simulink model "EKF_SIL_02_newdelIpsOOSM"  (R2015a)
settings: Solver=ode45  StartTime=0.0  StopTime=50  RelTol=1e-3
model workspace: external: MATLAB File InitOOSM.m (data not in the file)
values from neighbouring files (symbols this model uses):
  Cov_nu = [0.005 0 0 0 ... (first row only)    [InitOOSM.m]    (also in InitSIL.m; Init_Model_02_Simulink.m; Init_Model_02_Simulink_SIL1.m)
  Cov_r = [0.003 0 0 ... (first row only)    [InitOOSM.m]    (also in InitSIL.m; Init_Model_02_Simulink.m; Init_Model_02_Simulink_SIL1.m)
  e_force_x = 0    [InitOOSM.m]    (also in InitSIL.m; Init_Model_02_Simulink.m; Init_Model_02_Simulink_SIL1.m)
  e_force_y = 0    [InitOOSM.m]    (also in InitSIL.m; Init_Model_02_Simulink.m; Init_Model_02_Simulink_SIL1.m)
  e_force_z = 0    [InitOOSM.m]    (also in InitSIL.m; Init_Model_02_Simulink.m; Init_Model_02_Simulink_SIL1.m)
  ieps = [-0.7071;0;0;0.7071]    [InitOOSM.m]    (also in InitSIL.m; Init_Model_02_Simulink.m = [-0.7071; 0; 0; 0.7071]; Init_Model_02_Simulink_SIL1.m)
  ita = [0.5;0.5;0.5;0.5]    [InitOOSM.m]    (also in InitSIL.m; Init_Model_02_Simulink.m = [0.5; 0.5; 0.5; 0.5]; Init_Model_02_Simulink_SIL1.m)
  n = 0.00    (= 0)    [InitOOSM.m]    (also in InitSIL.m; Init_Model_02_Simulink.m; Init_Model_02_Simulink_SIL1.m)
  P_0 = 0.5*eye(18,18)    [InitOOSM.m]    (also in InitSIL.m = 0.05*eye(12,12); Init_Model_02_Simulink.m = 0.005*eye(12,12); Init_Model_02_Simulink_SIL1.m = 0.005*eye(12,12))
  P_k = Simulink.Signal    [InitOOSM.m]    (also in InitSIL.m; Init_Model_02_Simulink.m; Init_Model_02_Simulink_SIL1.m)
  p_x = 0.75    [InitOOSM.m]    (also in InitSIL.m; Init_Model_02_Simulink.m; Init_Model_02_Simulink_SIL1.m)
  p_y = 0.125    [InitOOSM.m]    (also in InitSIL.m; Init_Model_02_Simulink.m; Init_Model_02_Simulink_SIL1.m)
  p_z = -0.8    [InitOOSM.m]    (also in InitSIL.m; Init_Model_02_Simulink.m; Init_Model_02_Simulink_SIL1.m)
  parameter_gravitation = 3.986005E+14    (= 398600500000000)    [InitOOSM.m]    (also in InitSIL.m; Init_Model_02_Simulink.m; Init_Model_02_Simulink_SIL1.m)
  rho = [0.04;0;0.3]    [InitOOSM.m]    (also in InitSIL.m; Init_Model_02_Simulink.m = [0.04; 0; 0.3]; Init_Model_02_Simulink_SIL1.m)
  rho_c = [-0.00017;   -0.9780;   -0.1854]    [InitOOSM.m]    (also in InitSIL.m = [0.00036;   -0.9865;   -0.1854]; Init_Model_02_Simulink.m = [0.00036; -0.9865; -0.1854]; Init_Model_02_Simulink_SIL1.m = [0.00036;   -0.9865;   -0.1854])
  sig_f = 2E-6    (= 2e-06)    [InitOOSM.m]    (also in InitSIL.m; Init_Model_02_Simulink.m; Init_Model_02_Simulink_SIL1.m)
  sig_tau = 2.5E-5    (= 2.5e-05)    [InitOOSM.m]    (also in InitSIL.m; Init_Model_02_Simulink.m; Init_Model_02_Simulink_SIL1.m)
  t_delta = 0.2    [InitOOSM.m]    (also in InitSIL.m; Init_Model_02_Simulink.m; Init_Model_02_Simulink_SIL1.m)
  t_Kalman = 0.01    [InitOOSM.m]    (also in InitSIL.m; Init_Model_02_Simulink.m; Init_Model_02_Simulink_SIL1.m)
  t_RobotSense = 0.05    [InitOOSM.m]    (also in InitSIL.m; Init_Model_02_Simulink.m; Init_Model_02_Simulink_SIL1.m)
  tau_1 = 0    [InitOOSM.m]    (also in InitSIL.m; Init_Model_02_Simulink.m; Init_Model_02_Simulink_SIL1.m)
  tau_2 = 0    [InitOOSM.m]    (also in InitSIL.m; Init_Model_02_Simulink.m; Init_Model_02_Simulink_SIL1.m)
  tau_3 = 0    [InitOOSM.m]    (also in InitSIL.m; Init_Model_02_Simulink.m; Init_Model_02_Simulink_SIL1.m)
  U_n_d = Simulink.Signal    [InitOOSM.m]    (also in InitSIL.m; Init_Model_02_Simulink.m; Init_Model_02_Simulink_SIL1.m)
  X_a_0 = [0; 0; 0; 1; 0; 0; 0; 0; 0; 0; 0; 0; 0;0;0;0;0;0;0;1]    [InitOOSM.m]    (also in InitSIL.m = [0; 0; 0; 1; 0; 0; 0; 0; 0; 0; 0; 0; 0]; Init_Model_02_Simulink.m = [0;0;0;0.707000000000000;0.707000000000000;0.200000000000000; Init_Model_02_Simulink_SIL1.m = [0;0;0.707;0.707;0.2;-0.02;0.0001;0.02;-1.80;0.50;-0.05;0.00)
  x_k = Simulink.Signal    [InitOOSM.m]    (also in InitSIL.m; Init_Model_02_Simulink.m; Init_Model_02_Simulink_SIL1.m)
libraries: simulink x9, dspmtrx3 x4, aerolibtransform2 x2, visionsinks x1
(part 2 of 6)

== system EKF_SIL_02_newdelIpsOOSM/EKF/OOSM_KF ==
  "trig_cap " : Inport
  P_pre : Inport  Port=2
  X_a_\(k) : Inport  Port=3
  V : Inport  Port=4
  trig_meas : Inport  Port=5
  ts_meas : Inport  Port=6
  " X_d1" : Inport  Port=7
  " X_d2" : Inport  Port=8
  " X_d3" : Inport  Port=9
  Constant : Constant  Value=0
  IC : InitialCondition  Value=0
  IC1 : InitialCondition  Value=0
  OOSM_KF : Subsystem
  OOSM_enable : Subsystem
  Scope : Scope
      settings: YMin=0  YMax=1  SaveName=ScopeData7
  Scope1 : Scope
      settings: YMin=0  YMax=1  SaveName=ScopeData34
  Selector : Selector  InputPortWidth=6  Indices=[4:6]
  Subsystem : Subsystem
  U_n_d : Outport
  x_d : Outport  Port=2
  P_d : Outport  Port=3
  UF : Outport  Port=4
  Phi : Outport  Port=5
  OOSM_trig : Outport  Port=6
  wires:
  "trig_cap "/1 -> OOSM_enable/1("trig_cap ")
  Constant/1 -> OOSM_KF/1(del_t)
  OOSM_enable/2(reset_trigger) -> IC1/1
  IC1/1 -> OOSM_KF/2(reset_trigger)
  OOSM_enable/3("q_nominal ") -> OOSM_KF/3(q_nominal)
  OOSM_KF/1(U_n_d) -> U_n_d/1
  OOSM_KF/2(x_d) -> x_d/1
  OOSM_KF/3(P_d) -> P_d/1
  P_pre/1 -> OOSM_KF/4(P_pre(k))
  Subsystem/1(X_a(k+1)) -> OOSM_KF/5("x(k) ")
  V/1 -> Selector/1, OOSM_KF/6(V), Subsystem/2(V)
  OOSM_enable/4(ieps_nominal_out) -> OOSM_KF/7(ieps_nominal)
  OOSM_KF/4(UF) -> UF/1
  OOSM_KF/5(Phi) -> Phi/1
  trig_meas/1 -> OOSM_enable/2(trig_meas)
  OOSM_enable/1(Trigger) -> IC/1
  Selector/1 -> OOSM_enable/3(omega_robot)
  OOSM_enable/5(OOSM_trig) -> Scope1/1, OOSM_trig/1
  ts_meas/1 -> OOSM_enable/4(ts_meas)
  X_a_\(k)/1 -> Subsystem/1(X_a)
  IC/1 -> OOSM_KF/Enable, Scope/1
  " X_d1"/1 -> OOSM_KF/8(" X_d1")
  " X_d2"/1 -> OOSM_KF/9(" X_d2")
  " X_d3"/1 -> OOSM_KF/10(" X_d3")

== system EKF_SIL_02_newdelIpsOOSM/EKF/Predictor ==
  X_a(K) : Inport
  P_previous(k) : Inport  Port=2
  trigger : Inport  Port=3
  V : Inport  Port=4
  Create Bus [State Vector,X_a] : Subsystem
  Create Bus [State Vector,X_a]1 : Subsystem
  Create State error covariance (P) : Subsystem
  Delay : Delay  DelayLength=1  InitialCondition=0
  Display : Display
  Integrator : Subsystem
  X_a(k+1) : Outport
  P_current(k+1) : Outport  Port=2
  wires:
  Create Bus [State Vector,X_a]1/1(X_bus) -> Create State error covariance (P)/1(X_a)
  Create State error covariance (P)/1(P_current) -> P_current(k+1)/1
  P_previous(k)/1 -> Create State error covariance (P)/2(P_previous)
  trigger/1 -> Delay/1
  V/1 -> Create State error covariance (P)/3(V), Integrator/2(V)
  X_a(K)/1 -> Create Bus [State Vector,X_a]1/1(X), Integrator/1(X_a)
  Create Bus [State Vector,X_a]/1(X_bus) -> Display/1, X_a(k+1)/1
  Integrator/1(X_a(k+1)) -> Create Bus [State Vector,X_a]/1(X)

== system EKF_SIL_02_newdelIpsOOSM/EKF/Trigger logic ==
  timestamp_target : Inport
  meas : Inport  Port=2
  timestamp_robot : Inport  Port=3
  Bus Selector : BusSelector  OutputSignals=r_c,Mu
  Bus Selector1 : BusSelector  OutputSignals=rho_c,ieps
  Compare To Zero1 : simulink/Logic and Bit Operations/Compare To Zero  relop=>  OutDataTypeStr=boolean
  Compare To Zero2 : simulink/Logic and Bit Operations/Compare To Zero  relop=>  OutDataTypeStr=boolean
  Detect Increase : simulink/Logic and Bit Operations/Detect Increase  vinit=0  InputProcessing=Inherited  OutDataTypeStr=boolean
  Detect Increase1 : simulink/Logic and Bit Operations/Detect Increase  vinit=0  InputProcessing=Inherited  OutDataTypeStr=boolean
  Dot Product1 : DotProduct  InputSameDT=on  OutDataTypeStr=Inherit: Inherit via internal rule
  Dot Product2 : DotProduct  InputSameDT=on  OutDataTypeStr=Inherit: Inherit via internal rule
  Logical Operator1 : Logic  AllPortsSameDT=off  OutDataTypeStr=boolean
  Logical Operator2 : Logic  Operator=OR  AllPortsSameDT=off  OutDataTypeStr=boolean
  Logical Operator3 : Logic  AllPortsSameDT=off  OutDataTypeStr=boolean
  Math Function1 : Math  Operator=transpose  SaturateOnIntegerOverflow=on
  Math Function2 : Math  Operator=transpose  SaturateOnIntegerOverflow=on
  Mux : Mux  Inputs=2
  Mux1 : Mux  Inputs=2
  Scope : Scope
      settings: YMin=0  YMax=1  SaveName=ScopeData32
  "Trigger " : Outport
  "Trigger_1 " : Outport  Port=2
  "Trigger_2 " : Outport  Port=3
  ts_meas : Outport  Port=4
  wires:
  meas/1 -> Bus Selector1/1, Bus Selector/1
  Bus Selector/1 -> Mux/1  "<r_c>"
  Bus Selector/2 -> Mux/2  "<Mu>"
  Bus Selector1/1 -> Mux1/1  "<rho_c>"
  Bus Selector1/2 -> Mux1/2  "<ieps>"
  Math Function1/1 -> Dot Product1/2
  Mux/1 -> Dot Product1/1, Math Function1/1
  Mux1/1 -> Dot Product2/1, Math Function2/1
  Math Function2/1 -> Dot Product2/2
  Dot Product1/1 -> Compare To Zero1/1
  Dot Product2/1 -> Compare To Zero2/1
  Compare To Zero1/1 -> Logical Operator1/1
  timestamp_robot/1 -> Detect Increase1/1
  Detect Increase/1 -> Logical Operator1/2
  Detect Increase1/1 -> Logical Operator3/2
  Compare To Zero2/1 -> Logical Operator3/1
  Logical Operator3/1 -> Logical Operator2/2, "Trigger_2 "/1
  timestamp_target/1 -> ts_meas/1, Detect Increase/1
  Logical Operator2/1 -> Scope/1, "Trigger "/1
  Logical Operator1/1 -> Logical Operator2/1, "Trigger_1 "/1

== system EKF_SIL_02_newdelIpsOOSM/Plant/Dynamic Model (Differential equations) ==
  X_a(t) : Inport
  Bus Creator : BusCreator
  Constant : Constant  Value=[0]
  Constant1 : Constant  Value=zeros(3,1)
  "Orbital Dynamics " : Subsystem
  Quaternion Kinematics : Subsystem
  Rotational Dynamics : Subsystem
  Vector Concatenate : Concatenate
  n : Constant  Value=n
  omega : Selector  NumberOfDimensions=2  InputPortWidth=3  IndexOptions=Index vector (dialog),Index vector (dialog)  Indices=[5 6 7],1  OutputSizes=1,1
  p : Constant  Value=[p_x;p_y;p_z]
  parameter_gravitation : Constant  Value=parameter_gravitation
  q : Selector  NumberOfDimensions=2  InputPortWidth=3  IndexOptions=Index vector (dialog),Index vector (dialog)  Indices=[1 2 3 4],1  OutputSizes=1,1
  r : Selector  NumberOfDimensions=2  InputPortWidth=3  IndexOptions=Index vector (dialog),Index vector (dialog)  Indices=[8 9 10],1  OutputSizes=1,1
  r_dot : Selector  NumberOfDimensions=2  InputPortWidth=3  IndexOptions=Index vector (dialog),Index vector (dialog)  Indices=[11 12 13],1  OutputSizes=1,1
  X_a(t+1) : Outport
  wires:
  Constant/1 -> Vector Concatenate/2
  p/1 -> Rotational Dynamics/2(p)
  Vector Concatenate/1 -> Quaternion Kinematics/2(omega_rel)
  parameter_gravitation/1 -> "Orbital Dynamics "/2(Mu)
  n/1 -> "Orbital Dynamics "/3(n)
  Quaternion Kinematics/1(q_dot) -> Bus Creator/1  "q_dot"
  Rotational Dynamics/1(omega_dot) -> Bus Creator/2  "omega_dot"
  X_a(t)/1 -> q/1, omega/1, r_dot/1, r/1
  q/1 -> Quaternion Kinematics/1(q)
  omega/1 -> Rotational Dynamics/1(omega), Vector Concatenate/1
  r/1 -> "Orbital Dynamics "/1(r)
  r_dot/1 -> "Orbital Dynamics "/4("r_dot "), Bus Creator/3
  Bus Creator/1 -> X_a(t+1)/1
  Constant1/1 -> Bus Creator/4

== system EKF_SIL_02_newdelIpsOOSM/Plant/Initial Conditions (create bus) ==
  Bus Creator : BusCreator
  Bus Creator1 : BusCreator  Inputs=3
  Bus Creator2 : BusCreator  Inputs=3
  Bus Creator3 : BusCreator  Inputs=3
  Bus Creator4 : BusCreator
  Demux : Demux  Outputs=13
  Display : Display
  Initial conditions (Dynamic Model) : FromFile  FileName=X_a_0_Model_02_Static.mat  SampleTime=0
  Initial conditions (Dynamic Model)1 : FromFile  FileName=X_a_0_Model_02.mat  SampleTime=0
  "X_a(0) " : Outport
  wires:
  Initial conditions (Dynamic Model)/1 -> ?
  Demux/1 -> Bus Creator/1  "q_1"
  Demux/2 -> Bus Creator/2  "q_2"
  Demux/3 -> Bus Creator/3  "q_3"
  Demux/4 -> Bus Creator/4  "q_0"
  Demux/5 -> Bus Creator1/1  "omega_x"
  Demux/6 -> Bus Creator1/2  "omega_y"
  Demux/7 -> Bus Creator1/3  "omega_z"
  Demux/8 -> Bus Creator2/1  "r_x"
  Demux/9 -> Bus Creator2/2  "r_y"
  Demux/10 -> Bus Creator2/3  "r_z"
  Demux/11 -> Bus Creator3/1  "r_x_dot"
  Demux/12 -> Bus Creator3/2  "r_y_dot"
  Demux/13 -> Bus Creator3/3  "r_z_dot"
  Bus Creator/1 -> Bus Creator4/1  "q"
  Bus Creator1/1 -> Bus Creator4/2  "omega"
  Bus Creator2/1 -> Bus Creator4/3  "r"
  Bus Creator3/1 -> Bus Creator4/4  "r_dot"
  Bus Creator4/1 -> Display/1, "X_a(0) "/1  "X_a(0)"
  Initial conditions (Dynamic Model)1/1 -> Demux/1

== system EKF_SIL_02_newdelIpsOOSM/Plots and display/Create Measurements [Pose]1 ==
  q : Inport
  r : Inport  Port=2
  rho : Inport  Port=3
  ita : Inport  Port=4
  "rho_c " : Inport  Port=5
  "Create Measurements [Orientation] " : Subsystem
  Create Measurements [Position] : Subsystem
  Rate Transition : RateTransition
  Rate Transition1 : RateTransition
  Rate Transition2 : RateTransition
  r_c : Outport
  Mu : Outport  Port=2
  wires:
  q/1 -> "Create Measurements [Orientation] "/1(q), Create Measurements [Position]/2(q)
  r/1 -> Create Measurements [Position]/1(r)
  "Create Measurements [Orientation] "/1(Mu) -> Mu/1
  ita/1 -> Rate Transition1/1
  Create Measurements [Position]/1(r_c) -> r_c/1
  rho/1 -> Rate Transition2/1
  "rho_c "/1 -> Rate Transition/1
  Rate Transition/1 -> Create Measurements [Position]/4("rho_c ")
  Rate Transition1/1 -> "Create Measurements [Orientation] "/2("ita ")
  Rate Transition2/1 -> Create Measurements [Position]/3(rho)

== system EKF_SIL_02_newdelIpsOOSM/Plots and display/Create Measurements [Pose]2 ==
  q : Inport
  r : Inport  Port=2
  rho : Inport  Port=3
  ita : Inport  Port=4
  "rho_c " : Inport  Port=5
  ieps : Inport  Port=6
  "Create Measurements [Orientation] " : Subsystem
  Create Measurements [Position] : Subsystem
  Rate Transition : RateTransition
  Rate Transition1 : RateTransition
  Rate Transition2 : RateTransition
  r_c : Outport
  Mu : Outport  Port=2
  wires:
  Rate Transition2/1 -> Create Measurements [Position]/3(rho)
  Rate Transition1/1 -> "Create Measurements [Orientation] "/2("ita ")
  "rho_c "/1 -> Rate Transition/1
  rho/1 -> Rate Transition2/1
  Create Measurements [Position]/1(r_c) -> r_c/1
  ita/1 -> Rate Transition1/1
  "Create Measurements [Orientation] "/1(Mu) -> Mu/1
  r/1 -> Create Measurements [Position]/1(r)
  q/1 -> Create Measurements [Position]/2(q), "Create Measurements [Orientation] "/1(q)
  Rate Transition/1 -> Create Measurements [Position]/4("rho_c ")
  ieps/1 -> Create Measurements [Position]/5("ieps "), "Create Measurements [Orientation] "/3("ieps ")

== system EKF_SIL_02_newdelIpsOOSM/VREP_SIMULINK_LINK/Subsystem1 ==
  In1 : Inport
  In2 : Inport  Port=2
  In3 : Inport  Port=3
  In4 : Inport  Port=4
  Bus Creator : BusCreator
  Compare To Zero : simulink/Logic and Bit Operations/Compare To Zero  relop=<=  OutDataTypeStr=boolean
  Delay : Delay  DelayLength=1  InitialCondition=[0;1;0;0]
  Demux : Demux
  Display : Display
  Display1 : Display
  Display2 : Display
  Dot Product : DotProduct  InputSameDT=on  OutDataTypeStr=Inherit: Inherit via internal rule
  Gain : Gain  Gain=-1
  Mux : Mux
  Scope : Scope
      settings: YMin=0.95  YMax=1.05  SaveName=ScopeData21
  Switch : Switch  Criteria=u2 > Threshold
  Out2 : Outport
  wires:
  In1/1 -> Mux/1
  In2/1 -> Mux/2
  In3/1 -> Mux/3
  In4/1 -> Mux/4
  Mux/1 -> Gain/1, Switch/3, Dot Product/1  "Mu"
  Delay/1 -> Dot Product/2
  Dot Product/1 -> Scope/1, Display/1, Compare To Zero/1
  Compare To Zero/1 -> Switch/2
  Gain/1 -> Switch/1, Display1/1
  Switch/1 -> Delay/1, Demux/1, Display2/1
  Demux/1 -> Bus Creator/1  "Mu_1"
  Demux/2 -> Bus Creator/2  "Mu_2"
  Demux/3 -> Bus Creator/3  "Mu_3"
  Bus Creator/1 -> Out2/1
  Demux/4 -> Bus Creator/4  "Mu_0"

== system EKF_SIL_02_newdelIpsOOSM/VREP_SIMULINK_LINK/Subsystem3 ==
  In1 : Inport
  In2 : Inport  Port=2
  In3 : Inport  Port=3
  In4 : Inport  Port=4
  Bus Creator : BusCreator
  Compare To Zero : simulink/Logic and Bit Operations/Compare To Zero  relop=<=  OutDataTypeStr=boolean
  Delay : Delay  DelayLength=1  InitialCondition=[0;0;0;1]
  Demux : Demux
  Display : Display
  Display1 : Display
  Display2 : Display
  Dot Product : DotProduct  InputSameDT=on  OutDataTypeStr=Inherit: Inherit via internal rule
  Gain : Gain  Gain=-1
  Mux : Mux
  Scope : Scope
      settings: YMin=0.95  YMax=1.05  SaveName=ScopeData21
  Switch : Switch  Criteria=u2 > Threshold
  Out2 : Outport
  wires:
  In1/1 -> Mux/1
  In2/1 -> Mux/2
  In3/1 -> Mux/3
  In4/1 -> Mux/4
  Mux/1 -> Gain/1, Switch/3, Dot Product/1  "ieps"
  Delay/1 -> Dot Product/2
  Dot Product/1 -> Scope/1, Display/1, Compare To Zero/1
  Compare To Zero/1 -> Switch/2
  Gain/1 -> Switch/1, Display1/1
  Switch/1 -> Delay/1, Demux/1, Display2/1
  Demux/1 -> Bus Creator/1  "ieps_1"
  Demux/2 -> Bus Creator/2  "ieps_2"
  Demux/3 -> Bus Creator/3  "ieps_3"
  Bus Creator/1 -> Out2/1
  Demux/4 -> Bus Creator/4  "ieps_0"

== system EKF_SIL_02_newdelIpsOOSM/EKF/Control Signal/Create Jacobian [ee//b @ee] ==
  theta : Inport
  Interpreted MATLAB Function : MATLABFcn  MATLABFcn=J_1_bot
  Interpreted MATLAB Function1 : MATLABFcn  MATLABFcn=J_2_bot
  Interpreted MATLAB Function2 : MATLABFcn  MATLABFcn=J_3_bot
  Interpreted MATLAB Function3 : MATLABFcn  MATLABFcn=J_4_bot
  Interpreted MATLAB Function4 : MATLABFcn  MATLABFcn=J_5_bot
  Interpreted MATLAB Function5 : MATLABFcn  MATLABFcn=J_6_bot
  Math Function : Math  Operator=transpose  SaturateOnIntegerOverflow=on
  Matrix Concatenate : Concatenate  NumInputs=6  Mode=Multidimensional array  ConcatenateDimension=2
  J : Outport
  wires:
  Matrix Concatenate/1 -> J/1
  Interpreted MATLAB Function2/1 -> Matrix Concatenate/3
  Interpreted MATLAB Function/1 -> Matrix Concatenate/1
  Interpreted MATLAB Function3/1 -> Matrix Concatenate/4
  Interpreted MATLAB Function1/1 -> Matrix Concatenate/2
  Interpreted MATLAB Function5/1 -> Matrix Concatenate/6
  Interpreted MATLAB Function4/1 -> Matrix Concatenate/5
  theta/1 -> Math Function/1
  Math Function/1 -> Interpreted MATLAB Function2/1, Interpreted MATLAB Function1/1, Interpreted MATLAB Function/1, Interpreted MATLAB Function5/1, Interpreted MATLAB Function4/1, Interpreted MATLAB Function3/1

== system EKF_SIL_02_newdelIpsOOSM/EKF/Control Signal/Create Rotation Matrix 2 ==
  q : Inport
  Add : Sum
  Add5 : Sum  Inputs=+++
  Constant1 : Constant  Value=-1
  Create Skew Symmetric : Subsystem
  Gain : Gain  Gain=2
  Gain1 : Gain  Gain=2
  Gain2 : Gain  Gain=2
  I : Constant  Value=eye(3,3)
  Math Function : Math  Operator=square  SaturateOnIntegerOverflow=on
  Math Function1 : Math  Operator=transpose  SaturateOnIntegerOverflow=on
  Product1 : Product
  Product2 : Product
  Product3 : Product  Multiplication=Matrix(*)
  Selector2 : Selector  NumberOfDimensions=2  InputPortWidth=3  IndexOptions=Index vector (dialog),Index vector (dialog)  Indices=[1 2 3],1  OutputSizes=1,1
  Selector3 : Selector  NumberOfDimensions=2  InputPortWidth=3  IndexOptions=Index vector (dialog),Index vector (dialog)  Indices=[4],1  OutputSizes=1,1
  R : Outport
  wires:
  Gain/1 -> Add/1
  Math Function/1 -> Gain/1
  Constant1/1 -> Add/2
  Selector3/1 -> Product2/2, Math Function/1
  Add/1 -> Product1/1
  I/1 -> Product1/2
  Selector2/1 -> Math Function1/1, Product3/1, Create Skew Symmetric/1(vector)
  Gain2/1 -> Add5/1
  Product2/1 -> Add5/2
  Create Skew Symmetric/1(skew symmetric Matrix) -> Gain1/1
  Gain1/1 -> Product2/1
  Product1/1 -> Add5/3
  Math Function1/1 -> Product3/2
  Product3/1 -> Gain2/1
  Add5/1 -> R/1
  q/1 -> Selector3/1, Selector2/1

== system EKF_SIL_02_newdelIpsOOSM/EKF/Control Signal/SS to vector ==
  SS : Inport
  Gain1 : Gain  Gain=-1
  Gain4 : Gain  Gain=-1
  Mux1 : Mux  Inputs=3
  Selector1 : Selector  NumberOfDimensions=2  InputPortWidth=3  IndexOptions=Index vector (dialog),Index vector (dialog)  Indices=[1],[3]  OutputSizes=1,1
  Selector2 : Selector  NumberOfDimensions=2  InputPortWidth=3  IndexOptions=Index vector (dialog),Index vector (dialog)  Indices=[2],[3]  OutputSizes=1,1
  Selector3 : Selector  NumberOfDimensions=2  InputPortWidth=3  IndexOptions=Index vector (dialog),Index vector (dialog)  Indices=[1],[2]  OutputSizes=1,1
  vec : Outport
  wires:
  Gain4/1 -> Mux1/3
  Gain1/1 -> Mux1/1
  Selector3/1 -> Gain4/1
  Selector2/1 -> Gain1/1
  Mux1/1 -> vec/1
  Selector1/1 -> Mux1/2
  SS/1 -> Selector2/1, Selector3/1, Selector1/1

== system EKF_SIL_02_newdelIpsOOSM/EKF/Create Measurements [Pose]2/Create Measurements [Orientation]  ==
  q : Inport
  "ita " : Inport  Port=2
  "ieps " : Inport  Port=3
  Bus Creator : BusCreator
  Demux : Demux
  MATLAB Function : MATLAB Function  TreatAsAtomicUnit=on
  MATLAB Function1 : MATLAB Function  TreatAsAtomicUnit=on
  Product : Product  Multiplication=Matrix(*)
  Product1 : Product  Multiplication=Matrix(*)
  "flag " : Constant  Value=0
  Mu : Outport
  wires:
  Demux/4 -> Bus Creator/4
  Demux/3 -> Bus Creator/3
  Demux/2 -> Bus Creator/2
  Demux/1 -> Bus Creator/1
  "flag "/1 -> MATLAB Function1/2(flag), MATLAB Function/2(flag)
  MATLAB Function/1(CrossTensor) -> Product/1
  "ita "/1 -> MATLAB Function/1(q)
  Bus Creator/1 -> Mu/1  "Mu"
  q/1 -> Product/2
  Product/1 -> MATLAB Function1/1(q)
  MATLAB Function1/1(CrossTensor) -> Product1/1
  "ieps "/1 -> Product1/2
  Product1/1 -> Demux/1

== system EKF_SIL_02_newdelIpsOOSM/EKF/Create Measurements [Pose]2/Create Measurements [Position] ==
  r : Inport
  q : Inport  Port=2
  rho : Inport  Port=3
  "rho_c " : Inport  Port=4
  "ieps " : Inport  Port=5
  Add : Sum
  Add1 : Sum
  Bus Creator : BusCreator  Inputs=3
  "Create Rotation Matrix " : Subsystem
  Create Rotation Matrix 1 : Subsystem
  Demux : Demux  Outputs=3
  Product : Product  Multiplication=Matrix(*)
  Product1 : Product  Multiplication=Matrix(*)
  r_c : Outport
  wires:
  Demux/3 -> Bus Creator/3  "r_c_z"
  Demux/2 -> Bus Creator/2  "r_c_y"
  Demux/1 -> Bus Creator/1  "r_c_x"
  Product/1 -> Add/2
  "Create Rotation Matrix "/1(R) -> Product/1
  rho/1 -> Product/2
  q/1 -> "Create Rotation Matrix "/1(q)
  Bus Creator/1 -> r_c/1  "r_c"
  r/1 -> Add/1
  Create Rotation Matrix 1/1(R) -> Product1/1
  "rho_c "/1 -> Add1/2
  Add1/1 -> Demux/1
  Add/1 -> Product1/2
  "ieps "/1 -> Create Rotation Matrix 1/1(q)
  Product1/1 -> Add1/1

== system EKF_SIL_02_newdelIpsOOSM/EKF/Measurement Update/Create X from X_a ==
  X_a(k) : Inport
  q_nominal(k) : Inport  Port=2
  ieps_nominal : Inport  Port=3
  Bus Creator1 : BusCreator  Inputs=6
  Bus Selector3 : BusSelector  OutputSignals=q_est,omega,r,r_dot,rho_c,ieps
  Bus Selector5 : BusSelector  OutputSignals=q_est,ieps
  Create Bus [State Vector,X_a] : Subsystem
  Create Bus [State Vector] : Subsystem
  Create del_q [body] : Subsystem
  Create del_q [inertial] : Subsystem
  IC : InitialCondition  Value=[X_a_0]
  X(k) : Outport
  q(k) : Outport  Port=2
  ieps(k) : Outport  Port=3
  wires:
  Create Bus [State Vector,X_a]/1(X_bus) -> Bus Selector3/1, Bus Selector5/1
  Create del_q [body]/1(del_q) -> Bus Creator1/1  "del_q"
  Bus Selector3/2 -> Bus Creator1/2  "<omega>"
  Bus Selector3/3 -> Bus Creator1/3  "<r>"
  Bus Selector3/4 -> Bus Creator1/4  "<r_dot>"
  Bus Creator1/1 -> Create Bus [State Vector]/1(X)
  Bus Selector5/1 -> Create del_q [body]/1(q)  "<q_est>"
  Create Bus [State Vector]/1(X_bus) -> X(k)/1
  X_a(k)/1 -> IC/1
  IC/1 -> Create Bus [State Vector,X_a]/1(X)
  Bus Selector3/1 -> q(k)/1  "<q_est>"
  q_nominal(k)/1 -> Create del_q [body]/2(q_nominal)
  ieps_nominal/1 -> Create del_q [inertial]/2(q_nominal)
  Bus Selector5/2 -> Create del_q [inertial]/1(q)  "<ieps>"
  Bus Selector3/5 -> Bus Creator1/5  "<rho_c>"
  Create del_q [inertial]/1(del_q) -> Bus Creator1/6  "del_ieps"
  Bus Selector3/6 -> ieps(k)/1  "<ieps>"

== system EKF_SIL_02_newdelIpsOOSM/EKF/Measurement Update/Prune P ==
  P_in : Inport
  Constant : Constant  Value=2
  Constant1 : Constant  Value=1e-5*eye(18,18)
  Divide : Product  Inputs=*/
  Math Function : Math  Operator=transpose  SaturateOnIntegerOverflow=on
  Sum : Sum  Inputs=|++
  Sum1 : Sum  Inputs=|++
  P_out : Outport
  wires:
  P_in/1 -> Sum/2, Math Function/1
  Math Function/1 -> Sum/1
  Sum/1 -> Divide/1
  Constant/1 -> Divide/2
  Divide/1 -> Sum1/1
  Constant1/1 -> Sum1/2
  Sum1/1 -> P_out/1

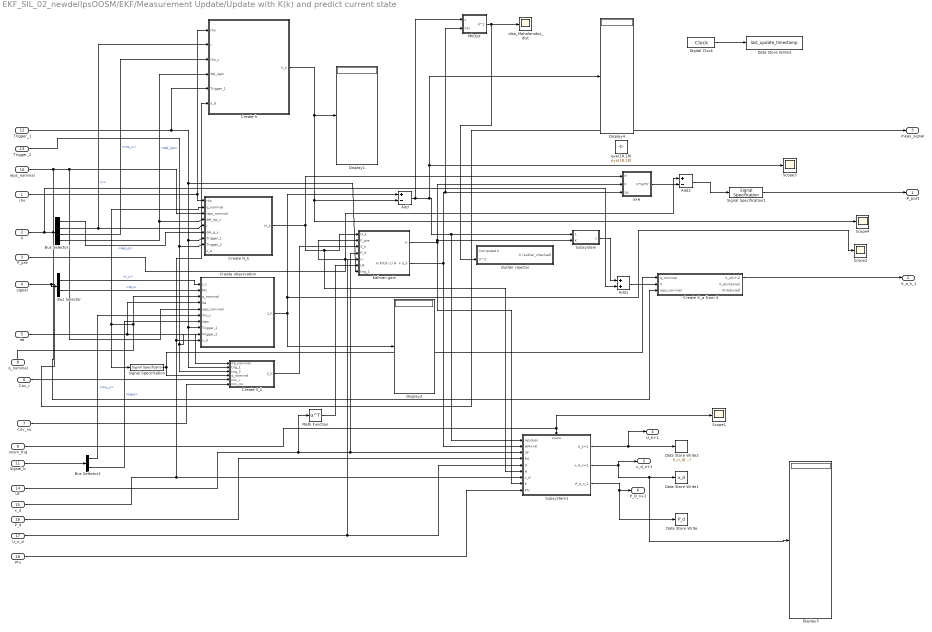
== system EKF_SIL_02_newdelIpsOOSM/EKF/Measurement Update/Update with K(k) and predict current state ==
  rho : Inport
  X : Inport  Port=2
  P_pre : Inport  Port=3
  signal : Inport  Port=4
  ita : Inport  Port=5
  Cov_r : Inport  Port=6
  Cov_nu : Inport  Port=7
  q_nominal : Inport  Port=8
  oosm_trig : Inport  Port=9
  ieps_nominal : Inport  Port=10
  Signal_b : Inport  Port=11
  Trigger_1 : Inport  Port=12
  Trigger_2 : Inport  Port=13
  UF : Inport  Port=14
  x_d : Inport  Port=15
  P_d : Inport  Port=16
  U_n_d : Inport  Port=17
  Phi : Inport  Port=18
  Add : Sum  Inputs=+-
  Add1 : Sum
  Add2 : Sum  Inputs=+-
  Bus Selector : BusSelector  OutputSignals=r_c,Mu
  Bus Selector1 : BusSelector  OutputSignals=del_q,r,rho_c,del_ips
  Bus Selector2 : BusSelector  OutputSignals=rho_c,ieps
  Create H_k : Subsystem
  Create S_k : Subsystem
  Create X_a from X : Subsystem
  Create h : Subsystem
  Create observation : Subsystem
  Data Store Write : DataStoreWrite  DataStoreName=P_d
  Data Store Write1 : DataStoreWrite  DialogController=Simulink.DDGSource  DataStoreName=x_d
  Data Store Write2 : DataStoreWrite  DataStoreName=U_n_d  DataStoreElements=U_n_d(:,:)
  Data Store Write3 : DataStoreWrite  DialogController=Simulink.DDGSource  DataStoreName=last_update_timestamp
  Digital Clock : DigitalClock  SampleTime=-1
  Display{1..4} (4 alike) : Display
  K*H : Subsystem
  Kalman gain : Subsystem
  Math Function : Math  Operator=transpose  SaturateOnIntegerOverflow=on
  MhDist : Subsystem
  Outlier rejector : Subsystem
  Scope{1..4} (4 alike) : Scope
      Scope1 settings: YMin=-0.35  YMax=0.3  SaveName=ScopeData19
      Scope2 settings: YMin=-1  YMax=1.75  SaveName=ScopeData28
      Scope3 settings: ShowLegends=on  TimeRange=40  YMin=-1  YMax=1.75  SaveName=ScopeData30
      Scope4 settings: YMin=-1  YMax=1.75  SaveName=ScopeData13
  Signal Specification : SignalSpecification  Dimensions=[4,1]
  Signal Specification1 : SignalSpecification  Dimensions=[18,18]
  Subsystem : Subsystem
  Subsystem1 : Subsystem
  disp_Mahalanobis_dist : Scope
      settings: TimeRange=100  YMin=0  YMax=32500  SaveName=ScopeData29
  eye(18,18) : Constant  Value=eye(18,18)
  P_post : Outport
  X_a_k_1 : Outport  Port=2
  meas_signal : Outport  Port=3
  U_K+1 : Outport  Port=4
  x_d_n+1 : Outport  Port=5
  P_D_n+1 : Outport  Port=6
  wires:
  Bus Selector/1 -> Create observation/1(r_c)  "<r_c>"
  Add/1 -> MhDist/1(x), Scope3/1, Display4/1, Subsystem1/1(residual), Subsystem/1(residual)
  Create observation/1(z_k) -> Scope2/1, Add/1, Display2/1
  Bus Selector1/2 -> Create H_k/5(r), Create h/2(r)  "<r>"
  Bus Selector1/1 -> Create H_k/6(del_q_v)  "<del_q>"
  Create H_k/1(H_k) -> K*H/1(H), Subsystem1/6(H), Kalman gain/1(H_k)
  P_pre/1 -> Add2/1, Kalman gain/2(P_pre)
  rho/1 -> Create h/1(rho), Create H_k/1(rho)
  Bus Selector/2 -> Create observation/2(Mu)  "<Mu>"
  Signal Specification/1 -> Create S_k/4(q_nominal), Create X_a from X/1(q_nominal)
  Add2/1 -> Signal Specification1/1
  Signal Specification1/1 -> P_post/1
  ita/1 -> Create S_k/1(ita_nominal), Create observation/4(ita)
  signal/1 -> meas_signal/1, Bus Selector/1
  q_nominal/1 -> Signal Specification/1, Create H_k/2(q_nominal), Create observation/3(q_nominal)
  Create X_a from X/1(X_a(k+1)) -> X_a_k_1/1
  Kalman gain/1(K) -> Subsystem1/8(K), Subsystem/2(K), K*H/2(K)
  Bus Selector1/3 -> Create h/3(rho_c)  "<rho_c>"
  Bus Selector1/4 -> Create h/4("del_ieps "), Create H_k/4(del_ips_v)  "<del_ips>"
  ieps_nominal/1 -> Create X_a from X/3(ieps_nominal), Create observation/5(ieps_nominal), Create H_k/3(ieps_nominal)
  Add1/1 -> Create X_a from X/2(X)
  X/1 -> Add1/2, Bus Selector1/1
  Signal_b/1 -> Bus Selector2/1
  Bus Selector2/1 -> Create observation/6(rho_c)  "<rho_c>"
  Bus Selector2/2 -> Create observation/7(ieps)  "<ieps>"
  Trigger_1/1 -> Kalman gain/7(trig_1), Create H_k/7(Trigger_1), Create S_k/2(trig_1), Create observation/8(Trigger_1), Create h/5(Trigger_1)
  Cov_r/1 -> Create S_k/5(cov_r)
  Cov_nu/1 -> Create S_k/6(cov_nu)
  Create S_k/1(S_k) -> Kalman gain/3(S_k)
  K*H/1(K*Sd*K') -> Add2/2
  Subsystem/1(K(z-h(x))) -> Add1/1
  MhDist/1(d^2) -> Outlier rejector/2(X^2), disp_Mahalanobis_dist/1
  Kalman gain/2(H.P(k|k-1).H' + S_k) -> Subsystem1/2(HPH+R), K*H/3(Sd), MhDist/2(Var)
  U_n_d/1 -> Kalman gain/5(U), Subsystem1/5(U)
  P_d/1 -> Subsystem1/4(Pd)
  x_d/1 -> Create observation/10(x_d), Create h/6(x_d), Subsystem1/7(x_d)
  Subsystem1/2(x_d_n+1) -> Data Store Write1/1, Display3/1, x_d_n+1/1
  Phi/1 -> Subsystem1/9(Phi)
  Trigger_2/1 -> Create H_k/8(Trigger_2), Create observation/9(Trigger_2), Create S_k/3(trig_2)
  oosm_trig/1 -> Subsystem1/Enable, Scope1/1
  Math Function/1 -> Kalman gain/6(UF)
  UF/1 -> Math Function/1, Subsystem1/3(UF), Kalman gain/4(P_d)
  Subsystem1/1(U_k+1) -> U_K+1/1, Data Store Write2/1
  Subsystem1/3(P_d_n_1) -> Data Store Write/1, P_D_n+1/1
  Create h/1(h_k) -> Scope4/1, Add/2, Display1/1
  Digital Clock/1 -> Data Store Write3/1

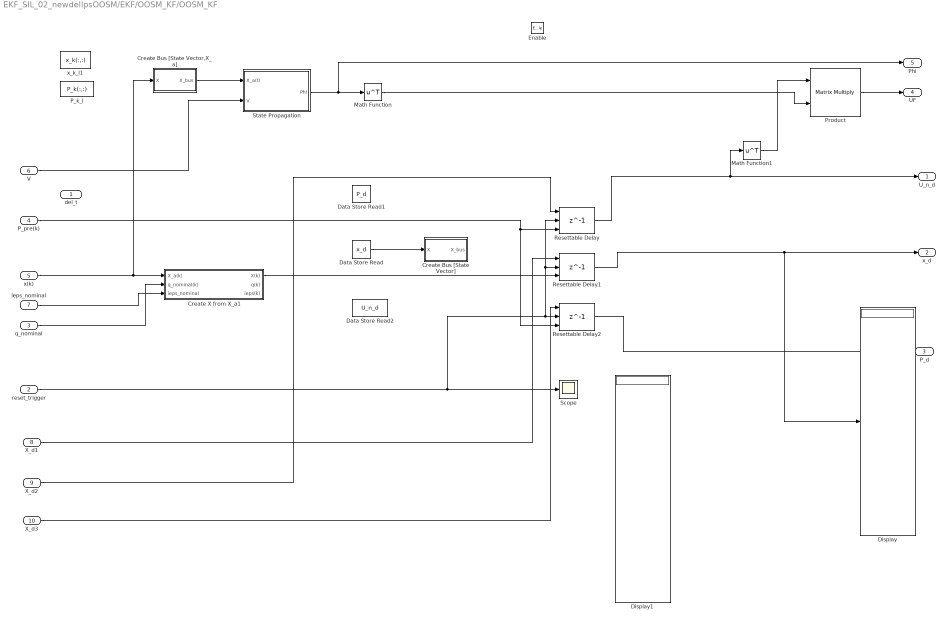
== system EKF_SIL_02_newdelIpsOOSM/EKF/OOSM_KF/OOSM_KF ==
  del_t : Inport
  reset_trigger : Inport  Port=2
  q_nominal : Inport  Port=3
  P_pre(k) : Inport  Port=4
  "x(k) " : Inport  Port=5
  V : Inport  Port=6
  ieps_nominal : Inport  Port=7
  " X_d1" : Inport  Port=8
  " X_d2" : Inport  Port=9
  " X_d3" : Inport  Port=10
  Enable : EnablePort
  Create Bus [State Vector,X_a] : Subsystem
  Create Bus [State Vector] : Subsystem
  Create X from X_a1 : Subsystem
  Data Store Read : DataStoreRead  DialogController=Simulink.DDGSource  DataStoreName=x_d
  Data Store Read1 : DataStoreRead  DataStoreName=P_d
  Data Store Read2 : DataStoreRead  DataStoreName=U_n_d
  Display : Display
  Display1 : Display
  Math Function : Math  Operator=transpose  SaturateOnIntegerOverflow=on
  Math Function1 : Math  Operator=transpose  SaturateOnIntegerOverflow=on
  P_k_l : DataStoreRead  DataStoreName=P_k  DataStoreElements=P_k(:,:)
  Product : Product  Multiplication=Matrix(*)
  Resettable Delay : Delay  DelayLength=1  InitialConditionSource=Input port  ExternalReset=Rising
      settings: InputPortMap=u0,r5,p4
  Resettable Delay1 : Delay  DelayLength=1  InitialConditionSource=Input port  ExternalReset=Rising
      settings: InputPortMap=u0,r5,p4
  Resettable Delay2 : Delay  DelayLength=1  InitialConditionSource=Input port  ExternalReset=Rising
      settings: InputPortMap=u0,r5,p4
  Scope : Scope
      settings: TimeRange=100  YMin=0  YMax=1  SaveName=ScopeData10
  State Propagation : Subsystem
  x_k_l1 : DataStoreRead  DataStoreName=x_k  DataStoreElements=x_k(:,:)
  U_n_d : Outport
  x_d : Outport  Port=2
  P_d : Outport  Port=3
  UF : Outport  Port=4
  Phi : Outport  Port=5
  wires:
  P_pre(k)/1 -> Resettable Delay/3, Resettable Delay2/3
  Resettable Delay1/1 -> Display/1, x_d/1
  reset_trigger/1 -> Resettable Delay/2, Resettable Delay1/2, Resettable Delay2/2, Scope/1
  Resettable Delay/1 -> Math Function1/1, U_n_d/1
  q_nominal/1 -> Create X from X_a1/2(q_nominal(k))
  "x(k) "/1 -> Create X from X_a1/1(X_a(k)), Create Bus [State Vector,X_a]/1(X)
  V/1 -> State Propagation/2(V)
  ieps_nominal/1 -> Create X from X_a1/3(ieps_nominal)
  Data Store Read/1 -> Create Bus [State Vector]/1(X)
  Math Function/1 -> Product/2
  Math Function1/1 -> Product/1
  Product/1 -> UF/1
  State Propagation/1(Phi) -> Phi/1, Math Function/1
  Create X from X_a1/1(X(k)) -> Resettable Delay1/3
  Create Bus [State Vector,X_a]/1(X_bus) -> State Propagation/1("X_a(t)\t")
  Resettable Delay2/1 -> P_d/1
  " X_d1"/1 -> Resettable Delay1/1
  " X_d2"/1 -> Resettable Delay/1
  " X_d3"/1 -> Resettable Delay2/1

== system EKF_SIL_02_newdelIpsOOSM/EKF/OOSM_KF/OOSM_enable ==
  "trig_cap " : Inport
  trig_meas : Inport  Port=2
  omega_robot : Inport  Port=3
  ts_meas : Inport  Port=4
  Chart : Stateflow chart  TreatAsAtomicUnit=on
  Chart1 : Stateflow chart  TreatAsAtomicUnit=on
  Create nominal q : Subsystem  TreatAsAtomicUnit=on
  Create nominal q2 : Subsystem  TreatAsAtomicUnit=on
  Data Store Write : DataStoreWrite  DialogController=Simulink.DDGSource  DataStoreName=q_nominal_d
  Data Store Write1 : DataStoreWrite  DialogController=Simulink.DDGSource  DataStoreName=ieps_nominal_d
  Delay1 : Delay  DelayLength=1  InitialCondition=0
  Digital Clock : DigitalClock  SampleTime=-1
  Display : Display
  Enabled Subsystem : Subsystem  TreatAsAtomicUnit=on
  Mux : Mux  Inputs=2
  Mux1 : Mux  Inputs=2
  Scope : Scope
      settings: YMin=0.95  YMax=1.05  SaveName=ScopeData16
  Scope1 : Scope
      settings: YMin=0.95  YMax=1.05  SaveName=ScopeData33
  Trigger : Outport
  reset_trigger : Outport  Port=2
  "q_nominal " : Outport  Port=3
  ieps_nominal_out : Outport  Port=4
  OOSM_trig : Outport  Port=5
  wires:
  Mux/1 -> Chart/Trigger
  "trig_cap "/1 -> Scope/1, reset_trigger/1, Mux1/2, Mux/2, Create nominal q2/Trigger, Create nominal q/Trigger  "camera_cap"
  Chart/1(out) -> Scope1/1, Trigger/1
  trig_meas/1 -> Delay1/1, Mux1/1  "meas_arrived"
  Create nominal q/1(q_nominal) -> Display/1, Data Store Write/1, "q_nominal "/1
  Create nominal q2/1(ieps_nominal) -> Data Store Write1/1, ieps_nominal_out/1
  Digital Clock/1 -> Create nominal q2/1(timestamp_meas)
  omega_robot/1 -> Create nominal q2/2(omega_robot)
  Mux1/1 -> Chart1/Trigger
  Chart1/1(out) -> OOSM_trig/1
  ts_meas/1 -> Create nominal q/1(timestamp_meas)
  Delay1/1 -> Mux/1

== system EKF_SIL_02_newdelIpsOOSM/EKF/OOSM_KF/Subsystem ==
  X_a : Inport
  V : Inport  Port=2
  Dynamic Model (Differential equations)2 : Subsystem
  Product : Product
  Sum : Sum  Inputs=|++
  t_Kalman : Constant  Value=t_Kalman
  X_a(k+1) : Outport
  wires:
  Dynamic Model (Differential equations)2/1(X_a_dot) -> Product/1
  t_Kalman/1 -> Product/2
  Product/1 -> Sum/1
  Sum/1 -> X_a(k+1)/1
  X_a/1 -> Sum/2, Dynamic Model (Differential equations)2/1(X_a(t))
  V/1 -> Dynamic Model (Differential equations)2/2("V ")

== system EKF_SIL_02_newdelIpsOOSM/EKF/Predictor/Create Bus [State Vector,X_a] ==
  X : Inport
  Bus Creator{1,3..5} (4 alike) : BusCreator  Inputs=3
  Bus Creator2 : BusCreator
  Bus Creator6 : BusCreator  Inputs=6
  Bus Creator7 : BusCreator
  Demux1 : Demux  Outputs=20
  X_bus : Outport
  wires:
  Bus Creator2/1 -> Bus Creator6/1  "q_est"
  Bus Creator3/1 -> Bus Creator6/2  "omega"
  Bus Creator4/1 -> Bus Creator6/3  "r"
  Bus Creator5/1 -> Bus Creator6/4  "r_dot"
  Bus Creator6/1 -> X_bus/1
  X/1 -> Demux1/1
  Demux1/1 -> Bus Creator2/1  "q_est_1"
  Demux1/2 -> Bus Creator2/2  "q_est_2"
  Demux1/3 -> Bus Creator2/3  "q_est_3"
  Demux1/4 -> Bus Creator2/4  "q_est_0"
  Demux1/5 -> Bus Creator3/1  "omega_x"
  Demux1/6 -> Bus Creator3/2  "omega_y"
  Demux1/7 -> Bus Creator3/3  "omega_z"
  Demux1/8 -> Bus Creator4/1  "r_x"
  Demux1/9 -> Bus Creator4/2  "r_y"
  Demux1/10 -> Bus Creator4/3  "r_z"
  Demux1/11 -> Bus Creator5/1  "r_x_dot"
  Demux1/12 -> Bus Creator5/2  "r_y_dot"
  Demux1/13 -> Bus Creator5/3  "r_z_dot"
  Demux1/14 -> Bus Creator1/1  "rho_c_x"
  Demux1/15 -> Bus Creator1/2  "rho_c_y"
  Demux1/16 -> Bus Creator1/3  "rho_c_z"
  Demux1/17 -> Bus Creator7/1  "ieps_1"
  Demux1/18 -> Bus Creator7/2  "ieps_2"
  Demux1/19 -> Bus Creator7/3  "ieps_3"
  Demux1/20 -> Bus Creator7/4  "ieps_0"
  Bus Creator1/1 -> Bus Creator6/5  "rho_c"
  Bus Creator7/1 -> Bus Creator6/6  "ieps"

== system EKF_SIL_02_newdelIpsOOSM/EKF/Predictor/Create Bus [State Vector,X_a]1 ==
  X : Inport
  Bus Creator{1,3..5} (4 alike) : BusCreator  Inputs=3
  Bus Creator2 : BusCreator
  Bus Creator6 : BusCreator  Inputs=6
  Bus Creator7 : BusCreator
  Demux1 : Demux  Outputs=20
  X_bus : Outport
  wires:
  Bus Creator2/1 -> Bus Creator6/1  "q_est"
  Bus Creator3/1 -> Bus Creator6/2  "omega"
  Bus Creator4/1 -> Bus Creator6/3  "r"
  Bus Creator5/1 -> Bus Creator6/4  "r_dot"
  Bus Creator6/1 -> X_bus/1
  X/1 -> Demux1/1
  Demux1/1 -> Bus Creator2/1  "q_est_1"
  Demux1/2 -> Bus Creator2/2  "q_est_2"
  Demux1/3 -> Bus Creator2/3  "q_est_3"
  Demux1/4 -> Bus Creator2/4  "q_est_0"
  Demux1/5 -> Bus Creator3/1  "omega_x"
  Demux1/6 -> Bus Creator3/2  "omega_y"
  Demux1/7 -> Bus Creator3/3  "omega_z"
  Demux1/8 -> Bus Creator4/1  "r_x"
  Demux1/9 -> Bus Creator4/2  "r_y"
  Demux1/10 -> Bus Creator4/3  "r_z"
  Demux1/11 -> Bus Creator5/1  "r_x_dot"
  Demux1/12 -> Bus Creator5/2  "r_y_dot"
  Demux1/13 -> Bus Creator5/3  "r_z_dot"
  Demux1/14 -> Bus Creator1/1  "rho_c_x"
  Demux1/15 -> Bus Creator1/2  "rho_c_y"
  Demux1/16 -> Bus Creator1/3  "rho_c_z"
  Demux1/17 -> Bus Creator7/1  "ieps_1"
  Demux1/18 -> Bus Creator7/2  "ieps_2"
  Demux1/19 -> Bus Creator7/3  "ieps_3"
  Demux1/20 -> Bus Creator7/4  "ieps_0"
  Bus Creator1/1 -> Bus Creator6/5  "rho_c"
  Bus Creator7/1 -> Bus Creator6/6  "ieps"

== system EKF_SIL_02_newdelIpsOOSM/EKF/Predictor/Create State error covariance (P) ==
  X_a : Inport
  P_previous : Inport  Port=2
  V : Inport  Port=3
  Add : Sum
  Math Function : Math  Operator=transpose  SaturateOnIntegerOverflow=on
  Matrix Concatenate : Concatenate  NumInputs=3  Mode=Multidimensional array  ConcatenateDimension=2
  Matrix Concatenate1 : Concatenate  NumInputs=3  Mode=Multidimensional array
  Matrix Concatenate2 : Concatenate  NumInputs=3  Mode=Multidimensional array  ConcatenateDimension=2
  Matrix Concatenate3 : Concatenate  NumInputs=3  Mode=Multidimensional array  ConcatenateDimension=2
  "Process Noise [Robot motion] " : Constant  Value=1e-6*eye(6,6)
  Process noise covariance [rotational] : Subsystem
  Process noise covariance [translational] : Subsystem
  Product : Product  Inputs=3  Multiplication=Matrix(*)
  State Propagation : Subsystem
  zeros(6,6) : Constant  Value=zeros(6,6)
  P_current : Outport
  wires:
  Math Function/1 -> Product/3
  P_previous/1 -> Product/2
  Add/1 -> P_current/1
  X_a/1 -> State Propagation/1("X_a(t)\t")
  Product/1 -> Add/2
  Matrix Concatenate2/1 -> Matrix Concatenate1/2
  Matrix Concatenate/1 -> Matrix Concatenate1/1
  zeros(6,6)/1 -> Matrix Concatenate/3, Matrix Concatenate/2, Matrix Concatenate2/3, Matrix Concatenate3/2, Matrix Concatenate3/1, Matrix Concatenate2/1
  State Propagation/1(Phi) -> Math Function/1, Product/1, Process noise covariance [rotational]/1(Phi)
  V/1 -> State Propagation/2(V)
  "Process Noise [Robot motion] "/1 -> Matrix Concatenate3/3
  Matrix Concatenate3/1 -> Matrix Concatenate1/3
  Matrix Concatenate1/1 -> Add/1
  Process noise covariance [rotational]/1(Q_r) -> Matrix Concatenate/1
  Process noise covariance [translational]/1(Q_t) -> Matrix Concatenate2/2

== system EKF_SIL_02_newdelIpsOOSM/EKF/Predictor/Integrator ==
  X_a : Inport
  V : Inport  Port=2
  Dynamic Model (Differential equations)2 : Subsystem
  Product : Product
  Sum : Sum  Inputs=|++
  t_Kalman : Constant  Value=t_Kalman
  X_a(k+1) : Outport
  wires:
  Dynamic Model (Differential equations)2/1(X_a_dot) -> Product/1
  t_Kalman/1 -> Product/2
  Product/1 -> Sum/1
  Sum/1 -> X_a(k+1)/1
  X_a/1 -> Sum/2, Dynamic Model (Differential equations)2/1(X_a(t))
  V/1 -> Dynamic Model (Differential equations)2/2("V ")

== system EKF_SIL_02_newdelIpsOOSM/Plant/Dynamic Model (Differential equations)/Orbital Dynamics  ==
  r : Inport
  Mu : Inport  Port=2
  n : Inport  Port=3
  "r_dot " : Inport  Port=4
  " " : Constant  Value=[0;0]
  Add : Sum
  Create Skew Symmetric : Subsystem
  Divide : Product  Inputs=*/
  Divide1 : Product  Inputs=*/
  Fcn : Fcn  Expr=u(1)^3
  Fcn1 : Fcn  Expr=u(1)^(1/3)
  Gain : Gain  Gain=-2
  Product : Product  Multiplication=Matrix(*)
  Product1 : Product  Multiplication=Matrix(*)
  Product2 : Product  Multiplication=Matrix(*)
  Product3 : Product
  Product4 : Product
  Product5 : Product
  Sum : Sum  Inputs=+--++
  Vector Concatenate1 : Concatenate
  "conc_re " : Constant  Value=[0;0]
  "e_force " : Constant  Value=[e_force_x;e_force_y;e_force_z]
  "norm " : Subsystem
  re : Concatenate
  "r_ddot " : Outport
  wires:
  " "/1 -> Vector Concatenate1/1
  Create Skew Symmetric/1(skew symmetric Matrix) -> Product/1, Product1/1, Product2/1
  Product1/1 -> Product2/2
  Mu/1 -> Product5/1, Divide/1
  Product/1 -> Gain/1
  "conc_re "/1 -> re/2
  re/1 -> Product4/1, Add/2
  Product5/1 -> Divide1/1
  "norm "/1("norm ") -> Fcn/1
  n/1 -> Product3/2, Vector Concatenate1/2, Product3/1
  Product3/1 -> Divide/2, Product4/2
  Vector Concatenate1/1 -> Create Skew Symmetric/1(vector)
  Add/1 -> "norm "/1(vector), Product5/2
  Gain/1 -> Sum/1
  Product2/1 -> Sum/2
  r/1 -> Product1/2, Add/1
  Product4/1 -> Sum/4
  "r_dot "/1 -> Product/2
  Divide1/1 -> Sum/3
  Fcn1/1 -> re/1
  Fcn/1 -> Divide1/2
  Divide/1 -> Fcn1/1
  "e_force "/1 -> Sum/5
  Sum/1 -> "r_ddot "/1

== system EKF_SIL_02_newdelIpsOOSM/Plant/Dynamic Model (Differential equations)/Quaternion Kinematics ==
  q : Inport
  omega_rel : Inport  Port=2
  Constant2 : Constant  Value=0.5
  MATLAB Function : MATLAB Function  TreatAsAtomicUnit=on
  Product : Product  Multiplication=Matrix(*)
  Product1 : Product
  flag : Constant
  q_dot : Outport
  wires:
  MATLAB Function/1(CrossTensor) -> Product/1
  flag/1 -> MATLAB Function/2(flag)
  Constant2/1 -> Product1/2
  q/1 -> MATLAB Function/1(q)
  omega_rel/1 -> Product/2
  Product1/1 -> q_dot/1
  Product/1 -> Product1/1

== system EKF_SIL_02_newdelIpsOOSM/Plant/Dynamic Model (Differential equations)/Rotational Dynamics ==
  omega : Inport
  p : Inport  Port=2
  Add : Sum
  Create  J : Subsystem
  Create Psi : Subsystem
  Product : Product  Multiplication=Matrix(*)
  tau : Constant  Value=[tau_1;tau_2;tau_3]
  omega_dot : Outport
  wires:
  omega/1 -> Create Psi/1("omega ")
  Create Psi/1(Psi) -> Add/1
  Add/1 -> omega_dot/1
  Product/1 -> Add/2
  p/1 -> Create Psi/2(p), Create  J/1(p)
  Create  J/1("J_k ") -> Product/1
  tau/1 -> Product/2

== system EKF_SIL_02_newdelIpsOOSM/Plots and display/Create Measurements [Pose]1/Create Measurements [Orientation]  ==
  q : Inport
  "ita " : Inport  Port=2
  Bus Creator : BusCreator
  Demux : Demux
  MATLAB Function : MATLAB Function  TreatAsAtomicUnit=on
  Product : Product  Multiplication=Matrix(*)
  "flag " : Constant  Value=0
  Mu : Outport
  wires:
  Product/1 -> Demux/1
  q/1 -> Product/2
  Bus Creator/1 -> Mu/1  "Mu"
  "ita "/1 -> MATLAB Function/1(q)
  MATLAB Function/1(CrossTensor) -> Product/1
  "flag "/1 -> MATLAB Function/2(flag)
  Demux/1 -> Bus Creator/1
  Demux/2 -> Bus Creator/2
  Demux/3 -> Bus Creator/3
  Demux/4 -> Bus Creator/4

== system EKF_SIL_02_newdelIpsOOSM/Plots and display/Create Measurements [Pose]1/Create Measurements [Position] ==
  r : Inport
  q : Inport  Port=2
  rho : Inport  Port=3
  "rho_c " : Inport  Port=4
  Add : Sum  Inputs=+++
  Bus Creator : BusCreator  Inputs=3
  "Create Rotation Matrix " : Subsystem
  Demux : Demux  Outputs=3
  Product : Product  Multiplication=Matrix(*)
  r_c : Outport
  wires:
  Add/1 -> Demux/1
  r/1 -> Add/2
  Bus Creator/1 -> r_c/1  "r_c"
  q/1 -> "Create Rotation Matrix "/1(q)
  "rho_c "/1 -> Add/1
  rho/1 -> Product/2
  "Create Rotation Matrix "/1(R) -> Product/1
  Product/1 -> Add/3
  Demux/1 -> Bus Creator/1  "r_c_x"
  Demux/2 -> Bus Creator/2  "r_c_y"
  Demux/3 -> Bus Creator/3  "r_c_z"

== system EKF_SIL_02_newdelIpsOOSM/Plots and display/Create Measurements [Pose]2/Create Measurements [Orientation]  ==
  q : Inport
  "ita " : Inport  Port=2
  "ieps " : Inport  Port=3
  Bus Creator : BusCreator
  Demux : Demux
  MATLAB Function : MATLAB Function  TreatAsAtomicUnit=on
  MATLAB Function1 : MATLAB Function  TreatAsAtomicUnit=on
  Product : Product  Multiplication=Matrix(*)
  Product1 : Product  Multiplication=Matrix(*)
  "flag " : Constant  Value=0
  Mu : Outport
  wires:
  Demux/4 -> Bus Creator/4
  Demux/3 -> Bus Creator/3
  Demux/2 -> Bus Creator/2
  Demux/1 -> Bus Creator/1
  "flag "/1 -> MATLAB Function1/2(flag), MATLAB Function/2(flag)
  MATLAB Function/1(CrossTensor) -> Product/1
  "ita "/1 -> MATLAB Function/1(q)
  Bus Creator/1 -> Mu/1  "Mu"
  q/1 -> Product/2
  Product/1 -> MATLAB Function1/1(q)
  MATLAB Function1/1(CrossTensor) -> Product1/1
  "ieps "/1 -> Product1/2
  Product1/1 -> Demux/1

== system EKF_SIL_02_newdelIpsOOSM/Plots and display/Create Measurements [Pose]2/Create Measurements [Position] ==
  r : Inport
  q : Inport  Port=2
  rho : Inport  Port=3
  "rho_c " : Inport  Port=4
  "ieps " : Inport  Port=5
  Add : Sum
  Add1 : Sum
  Bus Creator : BusCreator  Inputs=3
  "Create Rotation Matrix " : Subsystem
  Create Rotation Matrix 1 : Subsystem
  Demux : Demux  Outputs=3
  Product : Product  Multiplication=Matrix(*)
  Product1 : Product  Multiplication=Matrix(*)
  r_c : Outport
  wires:
  Demux/3 -> Bus Creator/3  "r_c_z"
  Demux/2 -> Bus Creator/2  "r_c_y"
  Demux/1 -> Bus Creator/1  "r_c_x"
  Product/1 -> Add/2
  "Create Rotation Matrix "/1(R) -> Product/1
  rho/1 -> Product/2
  q/1 -> "Create Rotation Matrix "/1(q)
  Bus Creator/1 -> r_c/1  "r_c"
  r/1 -> Add/1
  Create Rotation Matrix 1/1(R) -> Product1/1
  "rho_c "/1 -> Add1/2
  Add1/1 -> Demux/1
  Add/1 -> Product1/2
  "ieps "/1 -> Create Rotation Matrix 1/1(q)
  Product1/1 -> Add1/1

== system EKF_SIL_02_newdelIpsOOSM/EKF/Control Signal/Create Rotation Matrix 2/Create Skew Symmetric ==
  vector : Inport
  0 : Constant  Value=0
  Create 3x3 matrix : Subsystem
  Demux : Demux  Outputs=3
  Demux1 : Demux  Outputs=3
  Gain : Gain  Gain=-1
  skew symmetric Matrix : Outport
  wires:
  0/1 -> Create 3x3 matrix/1(a11), Create 3x3 matrix/9(a33), Create 3x3 matrix/5(a22)
  Demux/3 -> Create 3x3 matrix/2(a12)
  Demux1/2 -> Create 3x3 matrix/3(a13)
  Demux1/3 -> Create 3x3 matrix/4(a21)
  Demux/1 -> Create 3x3 matrix/6(a23)
  vector/1 -> Demux1/1, Gain/1
  Create 3x3 matrix/1(Matrix) -> skew symmetric Matrix/1
  Gain/1 -> Demux/1
  Demux/2 -> Create 3x3 matrix/7(a31)
  Demux1/1 -> Create 3x3 matrix/8(a32)

== system EKF_SIL_02_newdelIpsOOSM/EKF/Create Measurements [Pose]2/Create Measurements [Position]/Create Rotation Matrix  ==
  q : Inport
  Add : Sum
  Add5 : Sum  Inputs=+++
  Constant1 : Constant  Value=-1
  Create Skew Symmetric : Subsystem
  Gain : Gain  Gain=2
  Gain1 : Gain  Gain=2
  Gain2 : Gain  Gain=2
  I : Constant  Value=eye(3,3)
  Math Function : Math  Operator=square  SaturateOnIntegerOverflow=on
  Math Function1 : Math  Operator=transpose  SaturateOnIntegerOverflow=on
  Product1 : Product
  Product2 : Product
  Product3 : Product  Multiplication=Matrix(*)
  Selector2 : Selector  NumberOfDimensions=2  InputPortWidth=3  IndexOptions=Index vector (dialog),Index vector (dialog)  Indices=[1 2 3],1  OutputSizes=1,1
  Selector3 : Selector  NumberOfDimensions=2  InputPortWidth=3  IndexOptions=Index vector (dialog),Index vector (dialog)  Indices=[4],1  OutputSizes=1,1
  R : Outport
  wires:
  Gain/1 -> Add/1
  Math Function/1 -> Gain/1
  Constant1/1 -> Add/2
  Selector3/1 -> Product2/2, Math Function/1
  Add/1 -> Product1/1
  I/1 -> Product1/2
  Selector2/1 -> Math Function1/1, Product3/1, Create Skew Symmetric/1(vector)
  Gain2/1 -> Add5/1
  Product2/1 -> Add5/2
  Create Skew Symmetric/1(skew symmetric Matrix) -> Gain1/1
  Gain1/1 -> Product2/1
  Product1/1 -> Add5/3
  Math Function1/1 -> Product3/2
  Product3/1 -> Gain2/1
  Add5/1 -> R/1
  q/1 -> Selector3/1, Selector2/1

== system EKF_SIL_02_newdelIpsOOSM/EKF/Create Measurements [Pose]2/Create Measurements [Position]/Create Rotation Matrix 1 ==
  q : Inport
  Add : Sum
  Add5 : Sum  Inputs=+++
  Constant1 : Constant  Value=-1
  Create Skew Symmetric : Subsystem
  Gain : Gain  Gain=2
  Gain1 : Gain  Gain=2
  Gain2 : Gain  Gain=2
  I : Constant  Value=eye(3,3)
  Math Function : Math  Operator=square  SaturateOnIntegerOverflow=on
  Math Function1 : Math  Operator=transpose  SaturateOnIntegerOverflow=on
  Product1 : Product
  Product2 : Product
  Product3 : Product  Multiplication=Matrix(*)
  Selector2 : Selector  NumberOfDimensions=2  InputPortWidth=3  IndexOptions=Index vector (dialog),Index vector (dialog)  Indices=[1 2 3],1  OutputSizes=1,1
  Selector3 : Selector  NumberOfDimensions=2  InputPortWidth=3  IndexOptions=Index vector (dialog),Index vector (dialog)  Indices=[4],1  OutputSizes=1,1
  R : Outport
  wires:
  Gain/1 -> Add/1
  Math Function/1 -> Gain/1
  Constant1/1 -> Add/2
  Selector3/1 -> Product2/2, Math Function/1
  Add/1 -> Product1/1
  I/1 -> Product1/2
  Selector2/1 -> Math Function1/1, Product3/1, Create Skew Symmetric/1(vector)
  Gain2/1 -> Add5/1
  Product2/1 -> Add5/2
  Create Skew Symmetric/1(skew symmetric Matrix) -> Gain1/1
  Gain1/1 -> Product2/1
  Product1/1 -> Add5/3
  Math Function1/1 -> Product3/2
  Product3/1 -> Gain2/1
  Add5/1 -> R/1
  q/1 -> Selector3/1, Selector2/1

== system EKF_SIL_02_newdelIpsOOSM/EKF/Measurement Update/Create X from X_a/Create Bus [State Vector,X_a] ==
  X : Inport
  Bus Creator{1,3..5} (4 alike) : BusCreator  Inputs=3
  Bus Creator2 : BusCreator
  Bus Creator6 : BusCreator  Inputs=6
  Bus Creator7 : BusCreator
  Demux1 : Demux  Outputs=20
  X_bus : Outport
  wires:
  Bus Creator2/1 -> Bus Creator6/1  "q_est"
  Bus Creator3/1 -> Bus Creator6/2  "omega"
  Bus Creator4/1 -> Bus Creator6/3  "r"
  Bus Creator5/1 -> Bus Creator6/4  "r_dot"
  Bus Creator6/1 -> X_bus/1
  X/1 -> Demux1/1
  Demux1/1 -> Bus Creator2/1  "q_est_1"
  Demux1/2 -> Bus Creator2/2  "q_est_2"
  Demux1/3 -> Bus Creator2/3  "q_est_3"
  Demux1/4 -> Bus Creator2/4  "q_est_0"
  Demux1/5 -> Bus Creator3/1  "omega_x"
  Demux1/6 -> Bus Creator3/2  "omega_y"
  Demux1/7 -> Bus Creator3/3  "omega_z"
  Demux1/8 -> Bus Creator4/1  "r_x"
  Demux1/9 -> Bus Creator4/2  "r_y"
  Demux1/10 -> Bus Creator4/3  "r_z"
  Demux1/11 -> Bus Creator5/1  "r_x_dot"
  Demux1/12 -> Bus Creator5/2  "r_y_dot"
  Demux1/13 -> Bus Creator5/3  "r_z_dot"
  Demux1/14 -> Bus Creator1/1  "rho_c_x"
  Demux1/15 -> Bus Creator1/2  "rho_c_y"
  Demux1/16 -> Bus Creator1/3  "rho_c_z"
  Demux1/17 -> Bus Creator7/1  "ieps_1"
  Demux1/18 -> Bus Creator7/2  "ieps_2"
  Demux1/19 -> Bus Creator7/3  "ieps_3"
  Demux1/20 -> Bus Creator7/4  "ieps_0"
  Bus Creator1/1 -> Bus Creator6/5  "rho_c"
  Bus Creator7/1 -> Bus Creator6/6  "ieps"
